simulink model "symulinkModelWithAutotuner"  (R2022b)
settings: Solver=VariableStepAuto  StartTime=0.0  StopTime=5  RelTol=1e-3
values from neighbouring files (symbols this model uses):
  Ki = 2.14    [SystemGenerator.m]
  Kp = 0.14    [SystemGenerator.m]
  Ts = 0.01    [SystemGenerator.m]
undefined symbols (not defined in the file or in its folder): DiscIntNeverNeededParam, sigbuilder_block
libraries: slctrlblks x1, cstblocks x1
settings Model: Creator=corbi  LastModifiedBy=corbi

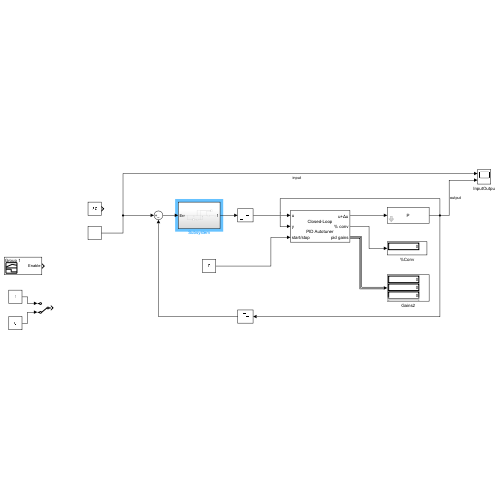
[thumbnail: Simulink's stored preview of the top-level diagram]
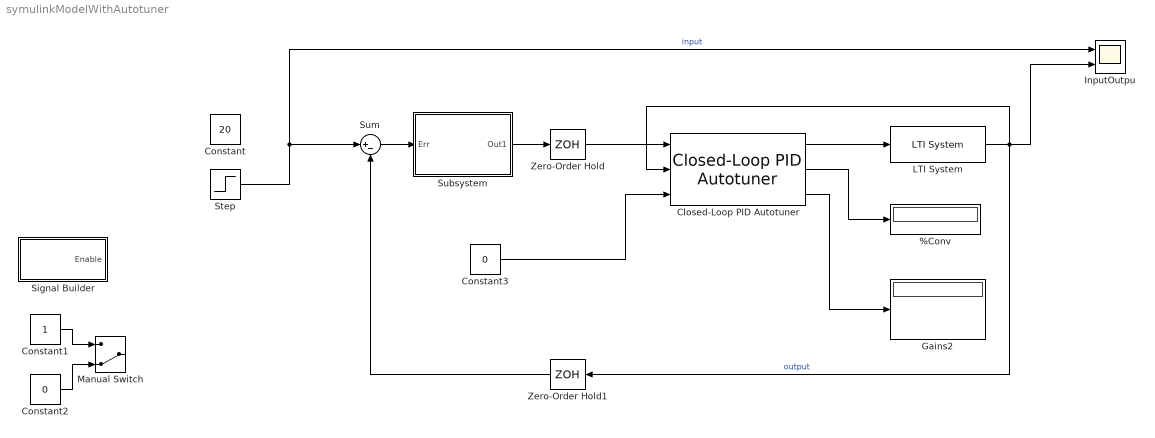
== system symulinkModelWithAutotuner ==
  %Conv : Display
  Closed-Loop PID Autotuner : slctrlblks/Closed-Loop PID Autotuner  PIDType=PI  PIDForm=Parallel  TimeDomain=continuous-time  DiscreteTs=0.01  TuningTs=0.2  UseTuningTs=off  IntegratorFormula=Forward Euler  FilterFormula=Forward Euler  ContinuousTs=0.01  Bandwidth=w_gc  UseExternalWC=off  TargetPM=phi_m  UseExternalPM=off  UseExternalAchievedPM=off  ExperimentMode=Superposition  PlantType=Stable  PlantSign=Positive  AmpSine=20  UseExternalAmpSine=off  UseExternalFRD=off  UseExternalU0=off  UseCompanion=off  NotDeployTuningModule=off  UsePLCCoder=off  OutputMode=control action + perturbation  BlockDataType=double  UseConnectedPID=on  blockpath=[]  tunedP=0  tunedI=0  tunedD=0  tunedN=100  tunedPM=0  EstimationWindowSize=3  UseExternalTuningParams=off  OutputChoice=VariantCandD  SingleMultiRateVariant=SingleSamplingRate  ExperimentModeVariant=VariantSuperimposed  NumEstimationPeriods=4  NumSettlingPeriods=2
  Constant : Constant  Value=20
  Constant1 : Constant
  Constant2 : Constant  Value=0
  Constant3 : Constant  Value=0
  Gains2 : Display
  InputOutpu : Scope  NumInputPorts=2
  LTI System : cstblocks/LTI System  sys=P  IC=[]
  Manual Switch : ManualSwitch  CurrentSetting=0
  Signal Builder : Subsystem  Tag=STV Subsys  LoadFcn=sigbuilder_block('load');  StartFcn=sigbuilder_block('start');  StopFcn=sigbuilder_block('stop');  ClipboardFcn=sigbuilder_block('clipboard');  mask(Sigbuilder block){tuvar=[0:10]}
      mask help: Simulink:masks:SigbuilderBlock_MD
      mask init:
      | if ~strcmp(get_param(bdroot(gcbh),'SimulationStatus'),'stopped') tuvar = sigbuilder_block('maskInit'); end
      settings: CopyFcn=sigbuilder_block('copy');  DeleteFcn=sigbuilder_block('delete');  ModelCloseFcn=sigbuilder_block('modelClose');  PreSaveFcn=sigbuilder_block('preSave');  PauseFcn=sigbuilder_block('pause');  ContinueFcn=sigbuilder_block('continue');  NameChangeFcn=sigbuilder_block('namechange');  OpenFcn=sigbuilder_block('open',[5.4 36 1141.2 516.6 ]);  CloseFcn=sigbuilder_block('close');
      mask Display: plot(0, 0, 100, 100,[2, 2, 32, 32, 2], [68, 8, 8, 68, 68],[32, 2], [38, 38], [32, 19, 2],[53, 60, 44], [32, 17, 17, 2],[16, 16, 31, 31]);txt = getActiveGroup(gcbh);text(2, 100, txt,'verticalAlignment', 'top');
  Step : Step  Time=2  After=20  SampleTime=Ts
  Subsystem : Subsystem
  Sum : Sum  Inputs=|+-
  Zero-Order Hold : ZeroOrderHold  SampleTime=Ts
  Zero-Order Hold1 : ZeroOrderHold  SampleTime=Ts
  wires:
  Constant3/1 -> Closed-Loop PID Autotuner/3
  Constant2/1 -> Manual Switch/2
  Constant1/1 -> Manual Switch/1
  Step/1 -> Sum/1, InputOutpu/1  "input"
  LTI System/1 -> Closed-Loop PID Autotuner/2, Zero-Order Hold1/1, InputOutpu/2  "output"
  Closed-Loop PID Autotuner/1 -> LTI System/1
  Closed-Loop PID Autotuner/2 -> %Conv/1
  Closed-Loop PID Autotuner/3 -> Gains2/1
  Subsystem/1(Out1) -> Zero-Order Hold/1
  Sum/1 -> Subsystem/1(Err)
  Zero-Order Hold/1 -> Closed-Loop PID Autotuner/1
  Zero-Order Hold1/1 -> Sum/2

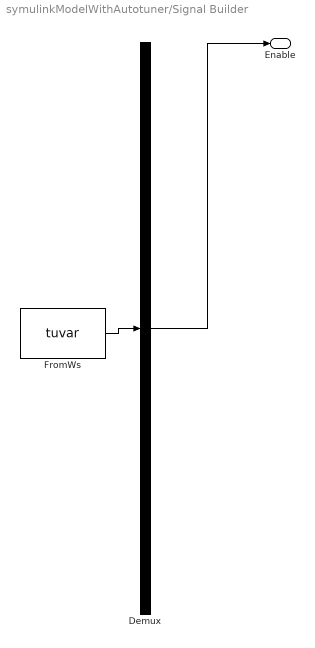
== system symulinkModelWithAutotuner/Signal Builder ==
  Demux : Demux  Tag=STV Demux  Outputs=1
      settings: DisplayOption=none
  FromWs : FromWorkspace  Tag=STV FromWs  VariableName=tuvar
      SigBuilderData=|
      | common.afterFinalStr = 'Extrapolate'
      | common.sampleTime = 0
      | dataSet.timeRange = [0 50]
      | dataSet.name = 'Group 1'
      | sbobj.Groups.Name = 'Group 1'
      | sbobj.Groups.Signals.Name = 'Enable'
      | sbobj.Groups.Signals.XData = [0 5 5 45 45 50]
      | sbobj.Groups.Signals.YData = [0 0 1 1 0 0]
      | sbobj.Groups.TimeRange = [0 50]
  Enable : Outport  Tag=STV Outport
  wires:
  FromWs/1 -> Demux/1
  Demux/1 -> Enable/1

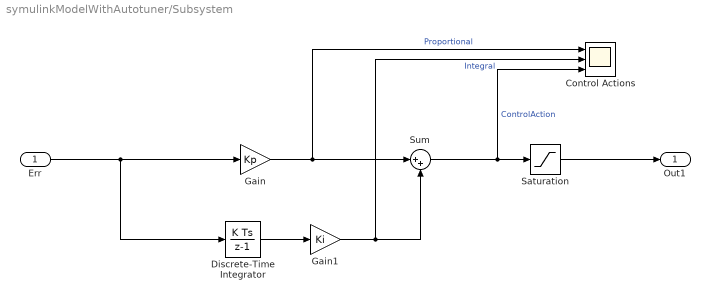
== system symulinkModelWithAutotuner/Subsystem ==
  Err : Inport
  Control Actions : Scope  NumInputPorts=3
  Discrete-Time Integrator : DiscreteIntegrator  SampleTime=Ts  ICPrevOutput=DiscIntNeverNeededParam  ICPrevScaledInput=DiscIntNeverNeededParam
  Gain : Gain  Gain=Kp
  Gain1 : Gain  Gain=Ki
  Saturation : Saturate  UpperLimit=8  LowerLimit=-8
  Sum : Sum  Inputs=|++
  Out1 : Outport
  wires:
  Err/1 -> Discrete-Time Integrator/1, Gain/1
  Gain/1 -> Control Actions/1, Sum/1  "Proportional"
  Discrete-Time Integrator/1 -> Gain1/1
  Sum/1 -> Control Actions/3, Saturation/1  "ControlAction"
  Gain1/1 -> Control Actions/2, Sum/2  "Integral"
  Saturation/1 -> Out1/1
